simulink model "dsm_l2_sim_deci_v2"  (R2025b)
settings: Solver=FixedStepDiscrete  StartTime=0.0  StopTime=1024  RelTol=1e-3  AbsTol=1e-6
values from neighbouring files (symbols this model uses):
  a1 = a(1)    [dsm_l1.m]    (also in dsm_o2_Simulink_HDLgeneration.m; dsm_o2_Simulink_compare.m; dsm_o2_Simulink_decimation.m; hodiewindow.m = 0.985371192726)
  a2 = a(2)    [dsm_l1.m]    (also in dsm_o2_Simulink_HDLgeneration.m; dsm_o2_Simulink_compare.m; dsm_o2_Simulink_decimation.m; hodiewindow.m = 0.49603771622)
  b1 = b(1)    [dsm_l1.m]    (also in dsm_o2_Simulink_HDLgeneration.m; dsm_o2_Simulink_compare.m; dsm_o2_Simulink_decimation.m; my_dsm_v1.m)
  c1 = c(1)    [dsm_l1.m]    (also in dsm_o2_Simulink_HDLgeneration.m; dsm_o2_Simulink_compare.m; dsm_o2_Simulink_decimation.m; my_dsm_v1.m)
  c2 = c(2)    [dsm_l1.m]    (also in dsm_o2_Simulink_HDLgeneration.m; dsm_o2_Simulink_compare.m; dsm_o2_Simulink_decimation.m; my_dsm_v1.m)
  DCFnum = Hdcf.Numerator    [decimation_filters.m]    (also in dsm_decimator_sim.m; dsm_l2_delsig_scmod2.m; dsm_o2_Simulink_HDLgeneration.m; dsm_o2_Simulink_decimation.m)
  fs = 1e6    (= 1000000)    [decimation_filters.m]    (also in dsm_decimator_sim.m; dsm_l1.m = 1; dsm_l1_dither.m = 1; dsm_l1_ntf.m = 1)
  Nsinc = 128    [decimation_filters.m]    (also in dsm_decimator_sim.m; dsm_l2_delsig_scmod2.m = 64; dsm_o2_Simulink_HDLgeneration.m; dsm_o2_Simulink_decimation.m)
  Ts = 1/fs    (= 1e-06)    [dsm_decimator_sim.m]    (also in dsm_l1.m = 1; dsm_l1_dither.m = 1; dsm_l1_ntf.m = 1; dsm_l1_sin.m = 1)
undefined symbols (not defined in the file or in its folder): dspblkCoreblockFVToolHelper, gcbh
libraries: dspmlti4 x3, dspsrcs4 x1
settings Model: Creator=mimeiners  LastModifiedBy=korvo
settings SolverCC: AutoScaleAbsTol=off  AlgebraicLoopSolver=TrustRegion
settings DataIOCC: ExternalInput=sigIn  LoadExternalInput=on  SaveFormat=Array  SignalLoggingSaveFormat=ModelDataLogs  ReturnWorkspaceOutputs=off  SignalLoggingName=sigsOut
settings OptimizationCC: BooleanDataType=off  ReuseModelBlockBuffer=off
settings DebuggingCC: SaveWithParameterizedLinksMsg=none  UnderspecifiedInitializationDetection=Classic  MergeDetectMultiDrivingBlocksExec=none  SignalResolutionControl=TryResolveAllWithWarning  MultiTaskDSMMsg=warning  MultiTaskCondExecSysMsg=none  UnconnectedInputMsg=warning  UnconnectedOutputMsg=warning  UnconnectedLineMsg=warning  ArithmeticOperatorsInVariantConditions=warning
settings HardwareCC: ProdBitPerPointer=32.0  ProdBitPerSizeT=32.0  ProdBitPerPtrDiffT=32.0  ProdLargestAtomicFloat=None  ProdIntDivRoundTo=Undefined  ProdEndianess=Unspecified  ProdWordSize=32.0  ProdHWDeviceType=32-bit Generic  TargetUnknown=on
settings ModelReferenceCC: EnableRefExpFcnMdlSchedulingChecks=on  PropagateSignalLabelsOutOfModel=off
settings SFSimCC: SimUseLocalCustomCode=off  CustomCodeUndefinedFunction=UseInterfaceOnly
settings RTWCC: TemplateMakefile=grt_vc.tmf  RTWUseLocalCustomCode=off  GPUComputeCapability=3.5  DLArmComputeVersion=19.05
settings GRTTargetCC: TargetLangStandard=C89/C90 (ANSI)  CombineOutputUpdateFcns=off  GRTInterface=on
settings ConfigComp: CovMetricSettings=dw  CovSaveCumulativeToWorkspaceVar=on  CovSaveSingleToWorkspaceVar=on  CovExternalEMLEnable=off

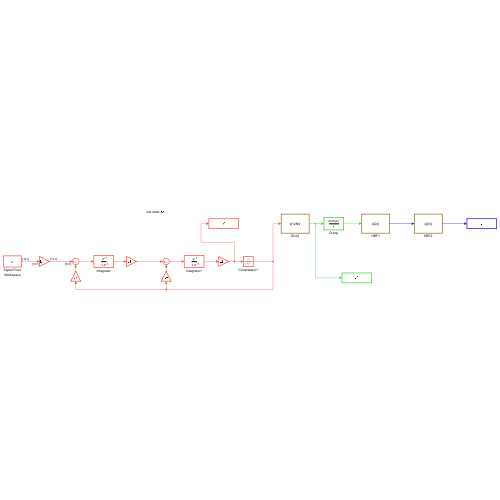
[thumbnail: Simulink's stored preview of the top-level diagram]
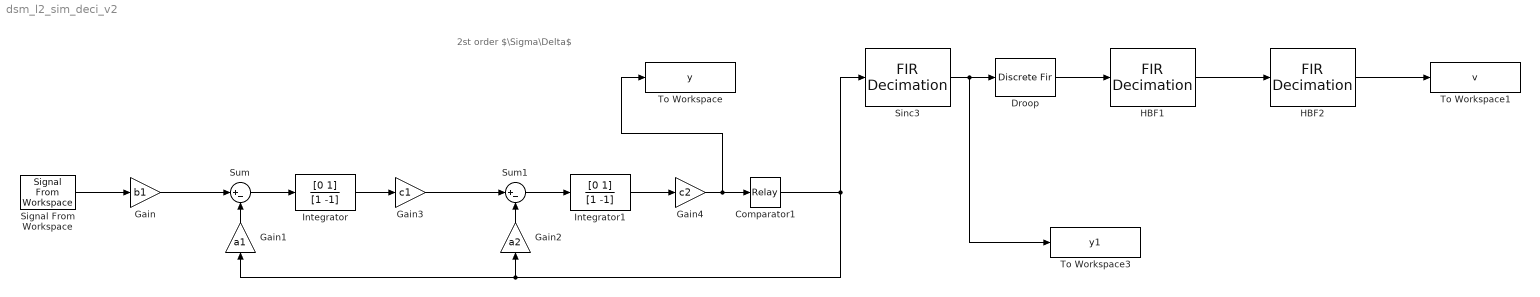
== system dsm_l2_sim_deci_v2 ==
  note: 2st order $\Sigma\Delta$
  Comparator1 : Relay  OffOutputValue=-1
  Droop : DiscreteFir  LoadFcn=dspblkCoreblockFVToolHelper(gcbh,'load');  Coefficients=DCFnum
      settings: CopyFcn=dspblkCoreblockFVToolHelper(gcbh,'copy');  DeleteFcn=dspblkCoreblockFVToolHelper(gcbh,'close');  ModelCloseFcn=dspblkCoreblockFVToolHelper(gcbh,'close');  PreSaveFcn=dspblkCoreblockFVToolHelper(gcbh,'presave');  PostSaveFcn=dspblkCoreblockFVToolHelper(gcbh,'postsave');  CloseFcn=dspblkCoreblockFVToolHelper(gcbh,'close');
  Gain : Gain  Gain=b1
  Gain1 : Gain  Gain=a1
  Gain2 : Gain  Gain=a2
  Gain3 : Gain  Gain=c1
  Gain4 : Gain  Gain=c2
  HBF1 : dspmlti4/FIR Decimation  FilterSource=Dialog parameters  h=HBF1num  D=2  filtStruct=Direct form  FilterObject=FDECIM  framing=Allow multirate processing  AllowArbitraryInputLength=off  inputOffset=0  outputBufInitCond=0  roundingMode=Floor  overflowMode=off  firstCoeffDataTypeStr=Inherit: Same word length as input  firstCoeffMin=[]  firstCoeffMax=[]  firstCoeffLastDataTypeStr=Inherit: Same word length as input  outputDataTypeStr=Inherit: Same as accumulator  outputMin=[]  outputMax=[]  outputLastDataTypeStr=Inherit: Same as accumulator
      settings: LibrarySourceBlock=|
      | dsphdlsupportfiltering/FIR
      | Decimation
  HBF2 : dspmlti4/FIR Decimation  FilterSource=Dialog parameters  h=HBF2num  D=2  filtStruct=Direct form  FilterObject=FDECIM  framing=Allow multirate processing  AllowArbitraryInputLength=off  inputOffset=0  outputBufInitCond=0  roundingMode=Floor  overflowMode=off  firstCoeffDataTypeStr=Inherit: Same word length as input  firstCoeffMin=[]  firstCoeffMax=[]  firstCoeffLastDataTypeStr=Inherit: Same word length as input  outputDataTypeStr=Inherit: Same as accumulator  outputMin=[]  outputMax=[]  outputLastDataTypeStr=Inherit: Same as accumulator
      settings: LibrarySourceBlock=|
      | dsphdlsupportfiltering/FIR
      | Decimation
  Integrator : DiscreteFilter  LoadFcn=dspblkCoreblockFVToolHelper(gcbh,'load');  Numerator=[0 1]  Denominator=[1 -1]  SampleTime=Ts
      settings: CopyFcn=dspblkCoreblockFVToolHelper(gcbh,'copy');  DeleteFcn=dspblkCoreblockFVToolHelper(gcbh,'close');  ModelCloseFcn=dspblkCoreblockFVToolHelper(gcbh,'close');  PreSaveFcn=dspblkCoreblockFVToolHelper(gcbh,'presave');  PostSaveFcn=dspblkCoreblockFVToolHelper(gcbh,'postsave');  CloseFcn=dspblkCoreblockFVToolHelper(gcbh,'close');
  Integrator1 : DiscreteFilter  LoadFcn=dspblkCoreblockFVToolHelper(gcbh,'load');  Numerator=[0 1]  Denominator=[1 -1]  SampleTime=Ts
      settings: CopyFcn=dspblkCoreblockFVToolHelper(gcbh,'copy');  DeleteFcn=dspblkCoreblockFVToolHelper(gcbh,'close');  ModelCloseFcn=dspblkCoreblockFVToolHelper(gcbh,'close');  PreSaveFcn=dspblkCoreblockFVToolHelper(gcbh,'presave');  PostSaveFcn=dspblkCoreblockFVToolHelper(gcbh,'postsave');  CloseFcn=dspblkCoreblockFVToolHelper(gcbh,'close');
  Signal From Workspace : dspsrcs4/Signal From Workspace  X=u  Ts=1/fs  nsamps=1  OutputAfterFinalValue=Setting to zero  ignoreOrWarnInputAndFrameLengths=off  OutputFrames=off
  Sinc3 : dspmlti4/FIR Decimation  FilterSource=Dialog parameters  h=hsinc3  D=Nsinc  filtStruct=Direct form  FilterObject=FDECIM  framing=Allow multirate processing  AllowArbitraryInputLength=off  inputOffset=0  outputBufInitCond=0  roundingMode=Floor  overflowMode=off  firstCoeffDataTypeStr=Inherit: Same word length as input  firstCoeffMin=[]  firstCoeffMax=[]  firstCoeffLastDataTypeStr=Inherit: Same word length as input  outputDataTypeStr=Inherit: Same as accumulator  outputMin=[]  outputMax=[]  outputLastDataTypeStr=Inherit: Same as accumulator
      settings: LibrarySourceBlock=|
      | dsphdlsupportfiltering/FIR
      | Decimation
  Sum : Sum  Inputs=|+-  InputSameDT=on  SaturateOnIntegerOverflow=on  OutDataTypeStr=Inherit: Same as first input
  Sum1 : Sum  Inputs=|+-  InputSameDT=on  SaturateOnIntegerOverflow=on  OutDataTypeStr=Inherit: Same as first input
  To Workspace : ToWorkspace  VariableName=y  SampleTime=-1
      settings: Save2DSignal=2-D array (concatenate along first dimension)
  To Workspace1 : ToWorkspace  VariableName=v  SampleTime=-1
      settings: Save2DSignal=2-D array (concatenate along first dimension)
  To Workspace3 : ToWorkspace  VariableName=y1  SampleTime=-1
      settings: Save2DSignal=2-D array (concatenate along first dimension)
  wires:
  Sum/1 -> Integrator/1
  Integrator/1 -> Gain3/1
  Signal From Workspace/1 -> Gain/1
  Gain3/1 -> Sum1/1
  Sum1/1 -> Integrator1/1
  Comparator1/1 -> Sinc3/1, Gain1/1, Gain2/1
  Integrator1/1 -> Gain4/1
  Gain/1 -> Sum/1
  Gain1/1 -> Sum/2
  Gain2/1 -> Sum1/2
  Gain4/1 -> To Workspace/1, Comparator1/1
  Sinc3/1 -> To Workspace3/1, Droop/1
  HBF1/1 -> HBF2/1
  HBF2/1 -> To Workspace1/1
  Droop/1 -> HBF1/1
